simulink model "CAMFC2_Pendulum_Comp_Lewis"  (R2018b)
settings: Solver=ode23  StartTime=0.0  StopTime=40  RelTol=1e-3  EnableMultiTasking=on
InitFcn:
  | constants_CAMFC2_Pendulum_Comp_Lewis
values from neighbouring files (symbols this model uses):
  AN = [     0 1 0 0 ... (first row only)    [constant_CAMFC2_01_WMR01.m]    (also in constant_CAMFC2_04_Comp.m = [     0 1 0 0 1; constant_CAMFC2_04_Quad_03.m; constant_CAMFC2_04_Simple.m; constant_CAMFC2_04_Simple_DoubleIntegrator.m)
  BN = [     1 0 0 0 ... (first row only)    [constant_CAMFC2_01_WMR01.m]    (also in constant_CAMFC2_04_Comp.m = [     0 0 0 0 0; constant_CAMFC2_04_Quad_03.m; constant_CAMFC2_04_Simple.m; constant_CAMFC2_04_Simple_DoubleIntegrator.m)
  Bp = 0.01    [constant_CAMFC2_04_Comp.m]    (also in constant_CAMFC2_04_Simple.m; constant_CAMFC2_04_Simple_DoubleIntegrator.m; constant_CAMFC2_04_Simple_DoubleIntegrator_02.m; constants_CAMFC2_Pendulum_Comp_Lewis.m)
  c = 2.2    [constants_CAMFC2_Pendulum_Comp_Lewis.m]
  Disturb_Freq = 2    [constant_CAMFC2_04_Comp.m]    (also in constant_CAMFC2_04_Simple.m; constant_CAMFC2_04_Simple_DoubleIntegrator.m; constant_CAMFC2_04_Simple_DoubleIntegrator_02.m; constants_CAMFC2_Pendulum_Comp_Lewis.m)
  Disturb_Val = 1    [constant_CAMFC2_04_Comp.m]    (also in constant_CAMFC2_04_Simple.m; constant_CAMFC2_04_Simple_DoubleIntegrator.m; constant_CAMFC2_04_Simple_DoubleIntegrator_02.m; constants_CAMFC2_Pendulum_Comp_Lewis.m)
  DN = [     1 0 0 0 ... (first row only)    [constant_CAMFC2_01_WMR01.m]    (also in constant_CAMFC2_04_Comp.m = [     2 0 0 0 0; constant_CAMFC2_04_Quad_03.m; constant_CAMFC2_04_Simple.m; constant_CAMFC2_04_Simple_DoubleIntegrator.m)
  F = 1.63    [constants_CAMFC2_Pendulum_Comp_Lewis.m]
  ge = 9.81    [constant_CAMFC2_04_Comp.m]    (also in constant_CAMFC2_04_Quad_03.m; constant_CAMFC2_04_Simple.m; constant_CAMFC2_04_Simple_DoubleIntegrator.m; constant_CAMFC2_04_Simple_DoubleIntegrator_02.m)
  Jp = 1    [constant_CAMFC2_04_Comp.m]    (also in constant_CAMFC2_04_Simple.m; constant_CAMFC2_04_Simple_DoubleIntegrator.m; constant_CAMFC2_04_Simple_DoubleIntegrator_02.m; constants_CAMFC2_Pendulum_Comp_Lewis.m)
  k = 1    [constants_CAMFC2_Pendulum_Comp_Lewis.m]
  k_NN = 1    [constants_CAMFC2_Pendulum_Comp_Lewis.m]
  lambda = 10    [constants_CAMFC2_Pendulum_Comp_Lewis.m]
  lp = 0.1    [constant_CAMFC2_04_Comp.m]    (also in constant_CAMFC2_04_Simple.m; constant_CAMFC2_04_Simple_DoubleIntegrator.m; constant_CAMFC2_04_Simple_DoubleIntegrator_02.m; constants_CAMFC2_Pendulum_Comp_Lewis.m)
  Mp = 0.1    [constant_CAMFC2_04_Comp.m]    (also in constant_CAMFC2_04_Simple.m; constant_CAMFC2_04_Simple_DoubleIntegrator.m; constant_CAMFC2_04_Simple_DoubleIntegrator_02.m; constants_CAMFC2_Pendulum_Comp_Lewis.m)
  N = 4    [constant_CAMFC2_01_WMR01.m]    (also in constant_CAMFC2_04_Comp.m = 5; constant_CAMFC2_04_Quad_03.m; constant_CAMFC2_04_Simple.m; constant_CAMFC2_04_Simple_DoubleIntegrator.m)
  n = 4    [constant_CAMFC2_01_WMR01.m]    (also in constant_CAMFC2_04_Comp.m = 2; constant_CAMFC2_04_Quad_03.m = 6; constant_CAMFC2_04_Simple.m = 2; constant_CAMFC2_04_Simple_DoubleIntegrator.m = 2)
  NN = 4    [constants_CAMFC2_Pendulum_Comp_Lewis.m]
  P = diag(p)    [constants_CAMFC2_Pendulum_Comp_Lewis.m]
settings Model: Creator=hp  LastModifiedBy=asafae
settings DataIOCC: LimitDataPoints=on  SaveFormat=Array
settings OptimizationCC: LifeSpan=inf
settings DebuggingCC: UnderspecifiedInitializationDetection=Classic  MergeDetectMultiDrivingBlocksExec=none  SolverPrmCheckMsg=warning  SFUnexpectedBacktrackingDiag=warning  SFNoUnconditionalDefaultTransitionDiag=warning  SFExecutionAtInitializationDiag=none
settings HardwareCC: ProdBitPerPointer=32  ProdBitPerSizeT=32  ProdBitPerPtrDiffT=32  ProdLargestAtomicFloat=None  ProdIntDivRoundTo=Undefined  ProdEndianess=Unspecified  ProdWordSize=32  ProdHWDeviceType=32-bit Generic
settings ModelReferenceCC: PropagateSignalLabelsOutOfModel=off
settings SFSimCC: SimUseLocalCustomCode=off
settings RTWCC: RTWUseLocalCustomCode=off
settings CodeAppCC: StateflowObjectComments=on
settings GRTTargetCC: TargetLangStandard=C89/C90 (ANSI)  GeneratePreprocessorConditionals=Disable all
settings ConfigComp: CovMetricSettings=dw  CovHtmlReporting=on  CovSaveCumulativeToWorkspaceVar=on  CovSaveSingleToWorkspaceVar=on  CovExternalEMLEnable=off

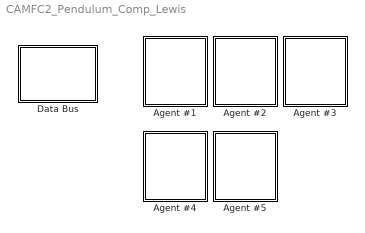
== system CAMFC2_Pendulum_Comp_Lewis ==
  Agent #1 : Subsystem
  Agent #2 : Subsystem
  Agent #3 : Subsystem
  Agent #4 : Subsystem
  Agent #5 : Subsystem
  "Data Bus " : Subsystem

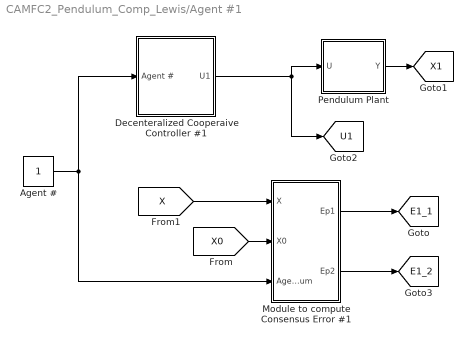
== system CAMFC2_Pendulum_Comp_Lewis/Agent #1 ==
  Agent # : Constant
  Decenteralized Cooperaive Controller #1 : Subsystem
  Module to compute Consensus Error #1 : MATLAB Function  TreatAsAtomicUnit=on
  Pendulum Plant : Subsystem
  tag scope: E1_1=global, E1_2=global, U1=global, X1=global
  wires:
  Agent #/1 -> Module to compute Consensus Error #1/3(Agent_Num), Decenteralized Cooperaive Controller #1/1(Agent #)
  Decenteralized Cooperaive Controller #1/1(U1) -> Pendulum Plant/1(U), [U1]
  [X0] -> Module to compute Consensus Error #1/2(X0)
  [X] -> Module to compute Consensus Error #1/1(X)
  Pendulum Plant/1(Y) -> [X1]
  Module to compute Consensus Error #1/1(Ep1) -> [E1_1]
  Module to compute Consensus Error #1/2(Ep2) -> [E1_2]

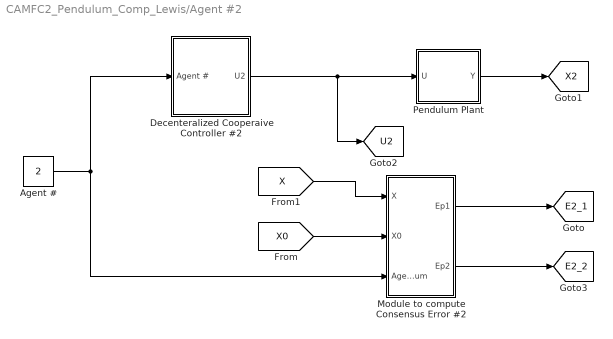
== system CAMFC2_Pendulum_Comp_Lewis/Agent #2 ==
  Agent # : Constant  Value=2
  Decenteralized Cooperaive Controller #2 : Subsystem
  Module to compute Consensus Error #2 : MATLAB Function  TreatAsAtomicUnit=on
  Pendulum Plant : Subsystem
  tag scope: E2_1=global, E2_2=global, U2=global, X2=global
  wires:
  Pendulum Plant/1(Y) -> [X2]
  [X] -> Module to compute Consensus Error #2/1(X)
  [X0] -> Module to compute Consensus Error #2/2(X0)
  Decenteralized Cooperaive Controller #2/1(U2) -> Pendulum Plant/1(U), [U2]
  Agent #/1 -> Decenteralized Cooperaive Controller #2/1(Agent #), Module to compute Consensus Error #2/3(Agent_Num)
  Module to compute Consensus Error #2/1(Ep1) -> [E2_1]
  Module to compute Consensus Error #2/2(Ep2) -> [E2_2]

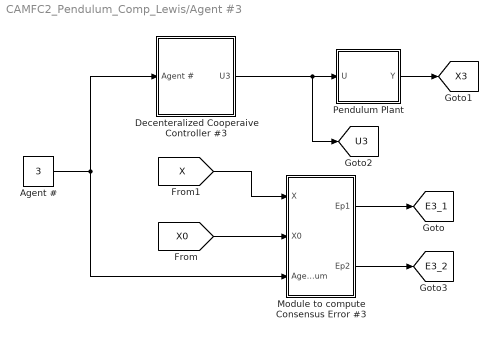
== system CAMFC2_Pendulum_Comp_Lewis/Agent #3 ==
  Agent # : Constant  Value=3
  Decenteralized Cooperaive Controller #3 : Subsystem
  Module to compute Consensus Error #3 : MATLAB Function  TreatAsAtomicUnit=on
  Pendulum Plant : Subsystem
  tag scope: E3_1=global, E3_2=global, U3=global, X3=global
  wires:
  Module to compute Consensus Error #3/2(Ep2) -> [E3_2]
  Module to compute Consensus Error #3/1(Ep1) -> [E3_1]
  Agent #/1 -> Module to compute Consensus Error #3/3(Agent_Num), Decenteralized Cooperaive Controller #3/1(Agent #)
  Decenteralized Cooperaive Controller #3/1(U3) -> Pendulum Plant/1(U), [U3]
  [X0] -> Module to compute Consensus Error #3/2(X0)
  [X] -> Module to compute Consensus Error #3/1(X)
  Pendulum Plant/1(Y) -> [X3]

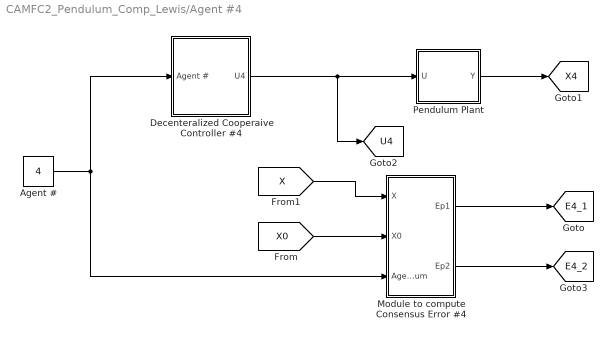
== system CAMFC2_Pendulum_Comp_Lewis/Agent #4 ==
  Agent # : Constant  Value=4
  Decenteralized Cooperaive Controller #4 : Subsystem
  Module to compute Consensus Error #4 : MATLAB Function  TreatAsAtomicUnit=on
  Pendulum Plant : Subsystem
  tag scope: E4_1=global, E4_2=global, U4=global, X4=global
  wires:
  Pendulum Plant/1(Y) -> [X4]
  [X] -> Module to compute Consensus Error #4/1(X)
  [X0] -> Module to compute Consensus Error #4/2(X0)
  Decenteralized Cooperaive Controller #4/1(U4) -> Pendulum Plant/1(U), [U4]
  Agent #/1 -> Decenteralized Cooperaive Controller #4/1(Agent #), Module to compute Consensus Error #4/3(Agent_Num)
  Module to compute Consensus Error #4/1(Ep1) -> [E4_1]
  Module to compute Consensus Error #4/2(Ep2) -> [E4_2]

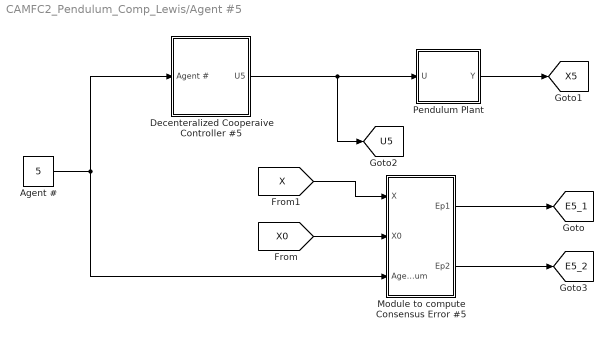
== system CAMFC2_Pendulum_Comp_Lewis/Agent #5 ==
  Agent # : Constant  Value=5
  Decenteralized Cooperaive Controller #5 : Subsystem
  Module to compute Consensus Error #5 : MATLAB Function  TreatAsAtomicUnit=on
  Pendulum Plant : Subsystem
  tag scope: E5_1=global, E5_2=global, U5=global, X5=global
  wires:
  Module to compute Consensus Error #5/2(Ep2) -> [E5_2]
  Module to compute Consensus Error #5/1(Ep1) -> [E5_1]
  Agent #/1 -> Module to compute Consensus Error #5/3(Agent_Num), Decenteralized Cooperaive Controller #5/1(Agent #)
  Decenteralized Cooperaive Controller #5/1(U5) -> Pendulum Plant/1(U), [U5]
  [X0] -> Module to compute Consensus Error #5/2(X0)
  [X] -> Module to compute Consensus Error #5/1(X)
  Pendulum Plant/1(Y) -> [X5]

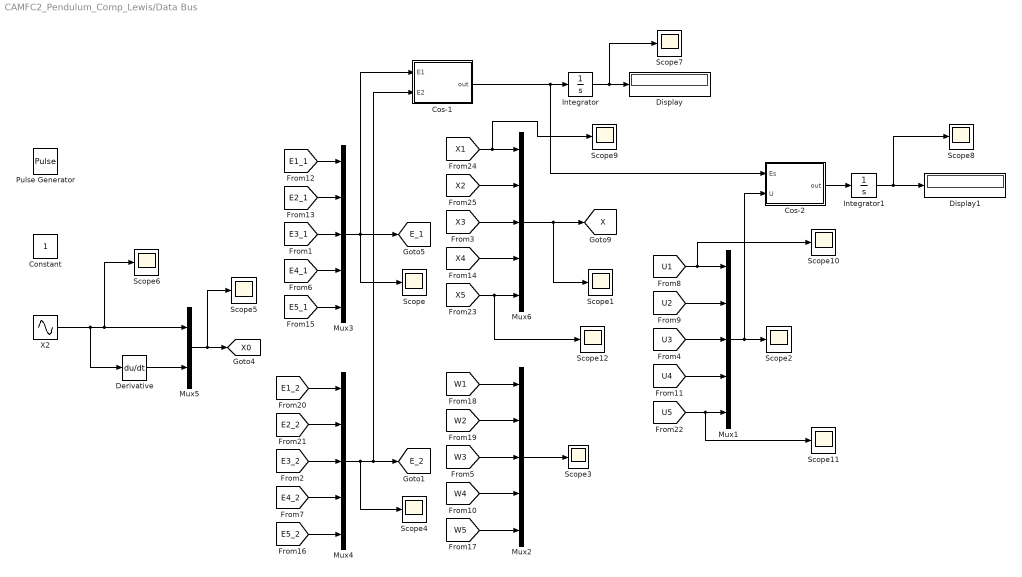
== system CAMFC2_Pendulum_Comp_Lewis/Data Bus  ==
  Constant : Constant
  Cos-1 : MATLAB Function  TreatAsAtomicUnit=on
  Cos-2 : MATLAB Function  TreatAsAtomicUnit=on
  Derivative : Derivative
  Display : Display
  Display1 : Display
  Integrator : Integrator
  Integrator1 : Integrator
  Mux{1..4,6} (5 alike) : Mux  Inputs=5
  Mux5 : Mux  Inputs=2
  Pulse Generator : DiscretePulseGenerator  PulseType=Time based  Amplitude=2  Period=20  PulseWidth=50
  Scope{,1..12} (13 alike) : Scope
  X2 : Sin  Amplitude=3  Frequency=0.5  SampleTime=0
  tag scope: E_1=global, E_2=global, X0=global, X=global
  wires:
  [E2_1] -> Mux3/2
  [E1_1] -> Mux3/1
  Mux3/1 -> Cos-1/1(E1), Scope/1, [E_1]
  [X2] -> Mux6/2
  [X1] -> Scope9/1, Mux6/1
  Mux6/1 -> Scope1/1, [X]
  [U2] -> Mux1/2
  [U1] -> Scope10/1, Mux1/1
  [W2] -> Mux2/2
  [W1] -> Mux2/1
  Mux2/1 -> Scope3/1
  [E2_2] -> Mux4/2
  [E1_2] -> Mux4/1
  Mux4/1 -> Cos-1/2(E2), [E_2], Scope4/1
  Mux5/1 -> Scope5/1, [X0]
  X2/1 -> Derivative/1, Scope6/1, Mux5/1
  Derivative/1 -> Mux5/2
  [E3_1] -> Mux3/3
  [E3_2] -> Mux4/3
  [X3] -> Mux6/3
  [U3] -> Mux1/3
  [W3] -> Mux2/3
  [E4_1] -> Mux3/4
  [E4_2] -> Mux4/4
  [W4] -> Mux2/4
  [U4] -> Mux1/4
  [X4] -> Mux6/4
  [E5_1] -> Mux3/5
  [E5_2] -> Mux4/5
  [W5] -> Mux2/5
  [U5] -> Scope11/1, Mux1/5
  [X5] -> Scope12/1, Mux6/5
  Cos-1/1(out) -> Cos-2/1(Es), Integrator/1
  Integrator/1 -> Scope7/1, Display/1
  Integrator1/1 -> Display1/1, Scope8/1
  Cos-2/1(out) -> Integrator1/1
  Mux1/1 -> Cos-2/2(U), Scope2/1

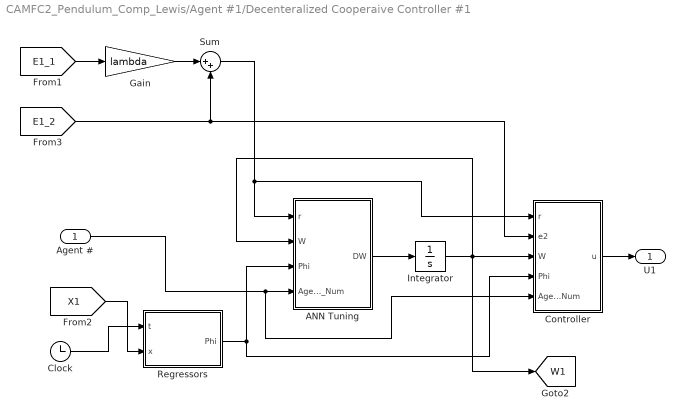
== system CAMFC2_Pendulum_Comp_Lewis/Agent #1/Decenteralized Cooperaive Controller #1 ==
  Agent # : Inport
  ANN Tuning : MATLAB Function  TreatAsAtomicUnit=on
  Clock : Clock
  Controller : MATLAB Function  TreatAsAtomicUnit=on
  Gain : Gain  Gain=lambda
  Integrator : Integrator  InitialCondition=zeros(NN,1)
  Regressors : MATLAB Function  TreatAsAtomicUnit=on
  Sum : Sum  Inputs=|++
  U1 : Outport
  tag scope: W1=global
  wires:
  ANN Tuning/1(DW) -> Integrator/1
  Integrator/1 -> ANN Tuning/2(W), [W1], Controller/3(W)
  Regressors/1(Phi) -> Controller/4(Phi), ANN Tuning/3(Phi)
  Agent #/1 -> Controller/5(Agent_Num), ANN Tuning/4(Agent_Num)
  Controller/1(u) -> U1/1
  Sum/1 -> Controller/1(r), ANN Tuning/1(r)
  [E1_2] -> Sum/2, Controller/2(e2)
  [E1_1] -> Gain/1
  Gain/1 -> Sum/1
  Clock/1 -> Regressors/1(t)
  [X1] -> Regressors/2(x)

== system CAMFC2_Pendulum_Comp_Lewis/Agent #1/Pendulum Plant ==
  U : Inport
  Plant : Subsystem
  Y : Outport
  wires:
  U/1 -> Plant/1(U)
  Plant/1(Y) -> Y/1

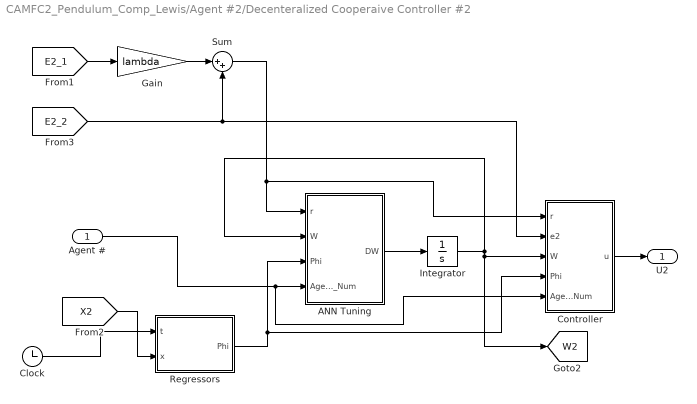
== system CAMFC2_Pendulum_Comp_Lewis/Agent #2/Decenteralized Cooperaive Controller #2 ==
  Agent # : Inport
  ANN Tuning : MATLAB Function  TreatAsAtomicUnit=on
  Clock : Clock
  Controller : MATLAB Function  TreatAsAtomicUnit=on
  Gain : Gain  Gain=lambda
  Integrator : Integrator  InitialCondition=zeros(NN,1)
  Regressors : MATLAB Function  TreatAsAtomicUnit=on
  Sum : Sum  Inputs=|++
  U2 : Outport
  tag scope: W2=global
  wires:
  Gain/1 -> Sum/1
  [E2_1] -> Gain/1
  [E2_2] -> Controller/2(e2), Sum/2
  Sum/1 -> Controller/1(r), ANN Tuning/1(r)
  Controller/1(u) -> U2/1
  Agent #/1 -> Controller/5(Agent_Num), ANN Tuning/4(Agent_Num)
  Regressors/1(Phi) -> Controller/4(Phi), ANN Tuning/3(Phi)
  Integrator/1 -> [W2], Controller/3(W), ANN Tuning/2(W)
  ANN Tuning/1(DW) -> Integrator/1
  Clock/1 -> Regressors/1(t)
  [X2] -> Regressors/2(x)

== system CAMFC2_Pendulum_Comp_Lewis/Agent #2/Pendulum Plant ==
  U : Inport
  Plant : Subsystem
  Y : Outport
  wires:
  U/1 -> Plant/1(U)
  Plant/1(Y) -> Y/1

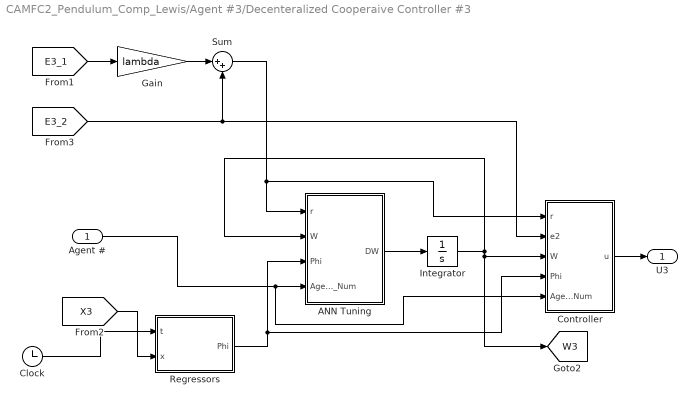
== system CAMFC2_Pendulum_Comp_Lewis/Agent #3/Decenteralized Cooperaive Controller #3 ==
  Agent # : Inport
  ANN Tuning : MATLAB Function  TreatAsAtomicUnit=on
  Clock : Clock
  Controller : MATLAB Function  TreatAsAtomicUnit=on
  Gain : Gain  Gain=lambda
  Integrator : Integrator  InitialCondition=zeros(NN,1)
  Regressors : MATLAB Function  TreatAsAtomicUnit=on
  Sum : Sum  Inputs=|++
  U3 : Outport
  tag scope: W3=global
  wires:
  ANN Tuning/1(DW) -> Integrator/1
  Integrator/1 -> ANN Tuning/2(W), Controller/3(W), [W3]
  Regressors/1(Phi) -> ANN Tuning/3(Phi), Controller/4(Phi)
  Agent #/1 -> ANN Tuning/4(Agent_Num), Controller/5(Agent_Num)
  Controller/1(u) -> U3/1
  Sum/1 -> ANN Tuning/1(r), Controller/1(r)
  [E3_2] -> Sum/2, Controller/2(e2)
  [E3_1] -> Gain/1
  Gain/1 -> Sum/1
  Clock/1 -> Regressors/1(t)
  [X3] -> Regressors/2(x)

== system CAMFC2_Pendulum_Comp_Lewis/Agent #3/Pendulum Plant ==
  U : Inport
  Plant : Subsystem
  Y : Outport
  wires:
  U/1 -> Plant/1(U)
  Plant/1(Y) -> Y/1

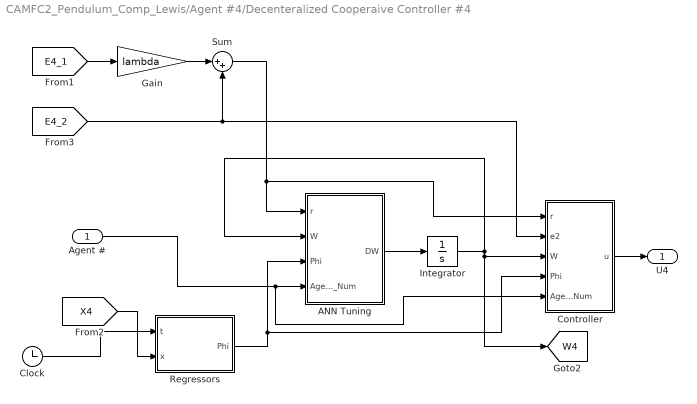
== system CAMFC2_Pendulum_Comp_Lewis/Agent #4/Decenteralized Cooperaive Controller #4 ==
  Agent # : Inport
  ANN Tuning : MATLAB Function  TreatAsAtomicUnit=on
  Clock : Clock
  Controller : MATLAB Function  TreatAsAtomicUnit=on
  Gain : Gain  Gain=lambda
  Integrator : Integrator  InitialCondition=zeros(NN,1)
  Regressors : MATLAB Function  TreatAsAtomicUnit=on
  Sum : Sum  Inputs=|++
  U4 : Outport
  tag scope: W4=global
  wires:
  Gain/1 -> Sum/1
  [E4_1] -> Gain/1
  [E4_2] -> Controller/2(e2), Sum/2
  Sum/1 -> Controller/1(r), ANN Tuning/1(r)
  Controller/1(u) -> U4/1
  Agent #/1 -> Controller/5(Agent_Num), ANN Tuning/4(Agent_Num)
  Regressors/1(Phi) -> Controller/4(Phi), ANN Tuning/3(Phi)
  Integrator/1 -> [W4], Controller/3(W), ANN Tuning/2(W)
  ANN Tuning/1(DW) -> Integrator/1
  Clock/1 -> Regressors/1(t)
  [X4] -> Regressors/2(x)

== system CAMFC2_Pendulum_Comp_Lewis/Agent #4/Pendulum Plant ==
  U : Inport
  Plant : Subsystem
  Y : Outport
  wires:
  U/1 -> Plant/1(U)
  Plant/1(Y) -> Y/1

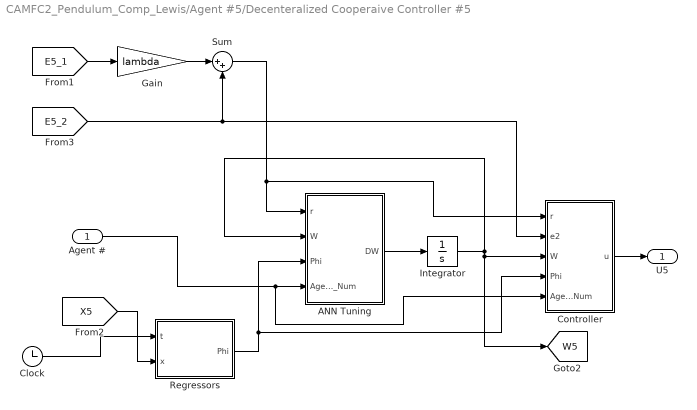
== system CAMFC2_Pendulum_Comp_Lewis/Agent #5/Decenteralized Cooperaive Controller #5 ==
  Agent # : Inport
  ANN Tuning : MATLAB Function  TreatAsAtomicUnit=on
  Clock : Clock
  Controller : MATLAB Function  TreatAsAtomicUnit=on
  Gain : Gain  Gain=lambda
  Integrator : Integrator  InitialCondition=zeros(NN,1)
  Regressors : MATLAB Function  TreatAsAtomicUnit=on
  Sum : Sum  Inputs=|++
  U5 : Outport
  tag scope: W5=global
  wires:
  ANN Tuning/1(DW) -> Integrator/1
  Integrator/1 -> ANN Tuning/2(W), Controller/3(W), [W5]
  Regressors/1(Phi) -> ANN Tuning/3(Phi), Controller/4(Phi)
  Agent #/1 -> ANN Tuning/4(Agent_Num), Controller/5(Agent_Num)
  Controller/1(u) -> U5/1
  Sum/1 -> ANN Tuning/1(r), Controller/1(r)
  [E5_2] -> Sum/2, Controller/2(e2)
  [E5_1] -> Gain/1
  Gain/1 -> Sum/1
  Clock/1 -> Regressors/1(t)
  [X5] -> Regressors/2(x)

== system CAMFC2_Pendulum_Comp_Lewis/Agent #5/Pendulum Plant ==
  U : Inport
  Plant : Subsystem
  Y : Outport
  wires:
  U/1 -> Plant/1(U)
  Plant/1(Y) -> Y/1

== system CAMFC2_Pendulum_Comp_Lewis/Agent #1/Pendulum Plant/Plant ==
  U : Inport
  Clock : Clock
  Integrator : Integrator
  Integrator1 : Integrator
  Mux : Mux  Inputs=2
  Plant : MATLAB Function  TreatAsAtomicUnit=on
  Scope3 : Scope
  Y : Outport
  wires:
  Plant/1(Dx1) -> Integrator/1
  Integrator/1 -> Plant/1(x1), Mux/1
  Integrator1/1 -> Plant/2(x2), Mux/2
  U/1 -> Plant/3(u)
  Plant/2(Dx2) -> Integrator1/1
  Clock/1 -> Plant/4(t)
  Mux/1 -> Y/1, Scope3/1

== system CAMFC2_Pendulum_Comp_Lewis/Agent #2/Pendulum Plant/Plant ==
  U : Inport
  Clock : Clock
  Integrator : Integrator  InitialCondition=-0.5
  Integrator1 : Integrator
  Mux : Mux  Inputs=2
  Plant : MATLAB Function  TreatAsAtomicUnit=on
  Scope3 : Scope
  Y : Outport
  wires:
  Plant/1(Dx1) -> Integrator/1
  Integrator/1 -> Plant/1(x1), Mux/1
  Integrator1/1 -> Plant/2(x2), Mux/2
  U/1 -> Plant/3(u)
  Plant/2(Dx2) -> Integrator1/1
  Clock/1 -> Plant/4(t)
  Mux/1 -> Y/1, Scope3/1

== system CAMFC2_Pendulum_Comp_Lewis/Agent #3/Pendulum Plant/Plant ==
  U : Inport
  Clock : Clock
  Integrator : Integrator  InitialCondition=+0.5
  Integrator1 : Integrator
  Mux : Mux  Inputs=2
  Plant : MATLAB Function  TreatAsAtomicUnit=on
  Scope3 : Scope
  Y : Outport
  wires:
  Plant/1(Dx1) -> Integrator/1
  Integrator/1 -> Plant/1(x1), Mux/1
  Integrator1/1 -> Plant/2(x2), Mux/2
  U/1 -> Plant/3(u)
  Plant/2(Dx2) -> Integrator1/1
  Clock/1 -> Plant/4(t)
  Mux/1 -> Y/1, Scope3/1

== system CAMFC2_Pendulum_Comp_Lewis/Agent #4/Pendulum Plant/Plant ==
  U : Inport
  Clock : Clock
  Integrator : Integrator  InitialCondition=-1
  Integrator1 : Integrator
  Mux : Mux  Inputs=2
  Plant : MATLAB Function  TreatAsAtomicUnit=on
  Scope3 : Scope
  Y : Outport
  wires:
  Plant/1(Dx1) -> Integrator/1
  Integrator/1 -> Plant/1(x1), Mux/1
  Integrator1/1 -> Plant/2(x2), Mux/2
  U/1 -> Plant/3(u)
  Plant/2(Dx2) -> Integrator1/1
  Clock/1 -> Plant/4(t)
  Mux/1 -> Y/1, Scope3/1

== system CAMFC2_Pendulum_Comp_Lewis/Agent #5/Pendulum Plant/Plant ==
  U : Inport
  Clock : Clock
  Integrator : Integrator  InitialCondition=+1
  Integrator1 : Integrator
  Mux : Mux  Inputs=2
  Plant : MATLAB Function  TreatAsAtomicUnit=on
  Scope3 : Scope
  Y : Outport
  wires:
  Plant/1(Dx1) -> Integrator/1
  Integrator/1 -> Plant/1(x1), Mux/1
  Integrator1/1 -> Plant/2(x2), Mux/2
  U/1 -> Plant/3(u)
  Plant/2(Dx2) -> Integrator1/1
  Clock/1 -> Plant/4(t)
  Mux/1 -> Y/1, Scope3/1

== matlab function CAMFC2_Pendulum_Comp_Lewis/Agent #2/Decenteralized Cooperaive Controller #2/ANN Tuning ==
  data: F parameter; r input; W input; Phi input; DW output; P parameter; DN parameter; BN parameter; k parameter; Agent_Num input
function DW = fcn(F,r,W,Phi, P, DN, BN, k,Agent_Num)

DW = -F * Phi * r' * P(Agent_Num,Agent_Num) * (DN(Agent_Num,Agent_Num)+BN(Agent_Num,Agent_Num)) - k * F * W;

end

== matlab function CAMFC2_Pendulum_Comp_Lewis/Agent #2/Decenteralized Cooperaive Controller #2/Controller ==
  data: u output size=1; r input; e2 input; W input; Phi input; Agent_Num input; c parameter; lambda parameter; BN parameter; DN parameter
function u = fcn(r,e2,W,Phi,Agent_Num, c, lambda, BN, DN)

u = (c*r) - (W' * Phi) + ( lambda / (DN(Agent_Num,Agent_Num)+BN(Agent_Num,Agent_Num)) * (e2) );

end

== matlab function CAMFC2_Pendulum_Comp_Lewis/Agent #2/Decenteralized Cooperaive Controller #2/Regressors ==
  data: t input; x input; Phi output; k_NN parameter; NN parameter
function Phi = fcn(t,x, k_NN, NN)

Phi = [(1/(1+exp(-k_NN*t)));(1/(1+exp(-k_NN*t)));(1/(1+exp(-k_NN*t)));(1/(1+exp(-k_NN*t)))]; %[1;x(1);(x(1)^2)];%;(x^3)];

end

== matlab function CAMFC2_Pendulum_Comp_Lewis/Agent #2/Module to compute Consensus Error #2 ==
  data: X input; X0 input; Ep1 output; AN parameter; BN parameter; N parameter; n parameter; Agent_Num input; Ep2 output
function [Ep1,Ep2] = fcn(X,X0,AN,BN,N,n,Agent_Num)

Xp1 = zeros(1,N);
Xp2 = zeros(1,N);
for i=1:N
    Xp1(1,i) = X((i-1)*n+1);
    Xp2(1,i) = X((i*n));
end

%% ---------------------------------------------------------------

Xp1_own = Xp1(1,Agent_Num);
Xp2_own = Xp2(1,Agent_Num);

Xp01 = X0(1);
Xp02 = X0(2);

Ep1 = ( BN(Agent_Num,Agent_Num)*(Xp01 - Xp1_own) );
Ep2 = ( BN(Agent_Num,Agent_Num)*(Xp02 - Xp2_own) );

for i=1:N        
    Xp1_other = Xp1(1,i);
    Xp2_other = Xp2(1,i);
    Ep1 = Ep1 + AN(Agent_Num,i)*(Xp1_other - Xp1_own);
    Ep2 = Ep2 + AN(Agent_Num,i)*(Xp2_other - Xp2_own);
end

end

== matlab function CAMFC2_Pendulum_Comp_Lewis/Agent #2/Pendulum Plant/Plant/Plant ==
  data: x1 input; Dx1 output; x2 input; Dx2 output; u input; t input; Jp parameter; Bp parameter; Mp parameter; ge parameter; lp parameter; Disturb_Val parameter; Disturb_Freq parameter
function [Dx1,Dx2]  = fcn(x1,x2,u,t,Jp, Bp, Mp, ge, lp, Disturb_Val, Disturb_Freq)

Dx1 = x2;
Dx2 = (1/Jp) * (u - Bp*x2 - Mp*ge*lp*sin(x1) + (Disturb_Val*sin(Disturb_Freq*t)));

end

== matlab function CAMFC2_Pendulum_Comp_Lewis/Agent #3/Decenteralized Cooperaive Controller #3/ANN Tuning ==
  data: F parameter; r input; W input; Phi input; DW output; P parameter; DN parameter; BN parameter; k parameter; Agent_Num input
function DW = fcn(F,r,W,Phi, P, DN, BN, k,Agent_Num)

DW = -F * Phi * r' * P(Agent_Num,Agent_Num) * (DN(Agent_Num,Agent_Num)+BN(Agent_Num,Agent_Num)) - k * F * W;

end

== matlab function CAMFC2_Pendulum_Comp_Lewis/Agent #3/Decenteralized Cooperaive Controller #3/Controller ==
  data: u output size=1; r input; e2 input; W input; Phi input; Agent_Num input; c parameter; lambda parameter; BN parameter; DN parameter
function u = fcn(r,e2,W,Phi,Agent_Num, c, lambda, BN, DN)

u = (c*r) - (W' * Phi) + ( lambda / (DN(Agent_Num,Agent_Num)+BN(Agent_Num,Agent_Num)) * (e2) );

end

== matlab function CAMFC2_Pendulum_Comp_Lewis/Agent #3/Decenteralized Cooperaive Controller #3/Regressors ==
  data: t input; x input; Phi output; k_NN parameter; NN parameter
function Phi = fcn(t,x, k_NN, NN)

Phi = [(1/(1+exp(-k_NN*t)));(1/(1+exp(-k_NN*t)));(1/(1+exp(-k_NN*t)));(1/(1+exp(-k_NN*t)))]; %[1;x(1);(x(1)^2)];%;(x^3)];

end

== matlab function CAMFC2_Pendulum_Comp_Lewis/Agent #3/Module to compute Consensus Error #3 ==
  data: X input; X0 input; Ep1 output; AN parameter; BN parameter; N parameter; n parameter; Agent_Num input; Ep2 output
function [Ep1,Ep2] = fcn(X,X0,AN,BN,N,n,Agent_Num)

Xp1 = zeros(1,N);
Xp2 = zeros(1,N);
for i=1:N
    Xp1(1,i) = X((i-1)*n+1);
    Xp2(1,i) = X((i*n));
end

%% ---------------------------------------------------------------

Xp1_own = Xp1(1,Agent_Num);
Xp2_own = Xp2(1,Agent_Num);

Xp01 = X0(1);
Xp02 = X0(2);

Ep1 = ( BN(Agent_Num,Agent_Num)*(Xp01 - Xp1_own) );
Ep2 = ( BN(Agent_Num,Agent_Num)*(Xp02 - Xp2_own) );

for i=1:N        
    Xp1_other = Xp1(1,i);
    Xp2_other = Xp2(1,i);
    Ep1 = Ep1 + AN(Agent_Num,i)*(Xp1_other - Xp1_own);
    Ep2 = Ep2 + AN(Agent_Num,i)*(Xp2_other - Xp2_own);
end

end

== matlab function CAMFC2_Pendulum_Comp_Lewis/Agent #3/Pendulum Plant/Plant/Plant ==
  data: x1 input; Dx1 output; x2 input; Dx2 output; u input; t input; Jp parameter; Bp parameter; Mp parameter; ge parameter; lp parameter; Disturb_Val parameter; Disturb_Freq parameter
function [Dx1,Dx2]  = fcn(x1,x2,u,t,Jp, Bp, Mp, ge, lp, Disturb_Val, Disturb_Freq)

Dx1 = x2;
Dx2 = (1/Jp) * (u - Bp*x2 - Mp*ge*lp*sin(x1) + (Disturb_Val*sin(Disturb_Freq*t)));

end

== matlab function CAMFC2_Pendulum_Comp_Lewis/Agent #4/Decenteralized Cooperaive Controller #4/ANN Tuning ==
  data: F parameter; r input; W input; Phi input; DW output; P parameter; DN parameter; BN parameter; k parameter; Agent_Num input
function DW = fcn(F,r,W,Phi, P, DN, BN, k,Agent_Num)

DW = -F * Phi * r' * P(Agent_Num,Agent_Num) * (DN(Agent_Num,Agent_Num)+BN(Agent_Num,Agent_Num)) - k * F * W;

end

== matlab function CAMFC2_Pendulum_Comp_Lewis/Agent #4/Decenteralized Cooperaive Controller #4/Controller ==
  data: u output size=1; r input; e2 input; W input; Phi input; Agent_Num input; c parameter; lambda parameter; BN parameter; DN parameter
function u = fcn(r,e2,W,Phi,Agent_Num, c, lambda, BN, DN)

u = (c*r) - (W' * Phi) + ( lambda / (DN(Agent_Num,Agent_Num)+BN(Agent_Num,Agent_Num)) * (e2) );

end

== matlab function CAMFC2_Pendulum_Comp_Lewis/Agent #4/Decenteralized Cooperaive Controller #4/Regressors ==
  data: t input; x input; Phi output; k_NN parameter; NN parameter
function Phi = fcn(t,x, k_NN, NN)

Phi = [(1/(1+exp(-k_NN*t)));(1/(1+exp(-k_NN*t)));(1/(1+exp(-k_NN*t)));(1/(1+exp(-k_NN*t)))]; %[1;x(1);(x(1)^2)];%;(x^3)];

end

== matlab function CAMFC2_Pendulum_Comp_Lewis/Agent #1/Decenteralized Cooperaive Controller #1/Controller ==
  data: u output size=1; r input; e2 input; W input; Phi input; Agent_Num input; c parameter; lambda parameter; BN parameter; DN parameter
function u = fcn(r,e2,W,Phi,Agent_Num, c, lambda, BN, DN)

u = (c*r) - (W' * Phi) + ( lambda / (DN(Agent_Num,Agent_Num)+BN(Agent_Num,Agent_Num)) * e2 );

end

== matlab function CAMFC2_Pendulum_Comp_Lewis/Agent #1/Decenteralized Cooperaive Controller #1/ANN Tuning ==
  data: F parameter; r input; W input; Phi input; DW output; P parameter; DN parameter; BN parameter; k parameter; Agent_Num input
function DW = fcn(F,r,W,Phi, P, DN, BN, k,Agent_Num)

DW = -F * Phi * r' * P(Agent_Num,Agent_Num) * (DN(Agent_Num,Agent_Num)+BN(Agent_Num,Agent_Num)) - k * F * W;

end

== matlab function CAMFC2_Pendulum_Comp_Lewis/Agent #1/Decenteralized Cooperaive Controller #1/Regressors ==
  data: t input; x input; Phi output; k_NN parameter; NN parameter
function Phi = fcn(t,x, k_NN, NN)

Phi = [(1/(1+exp(-k_NN*t)));(1/(1+exp(-k_NN*t)));(1/(1+exp(-k_NN*t)));(1/(1+exp(-k_NN*t)))]; %[1;x(1);(x(1)^2)];%;(x^3)];

end

== matlab function CAMFC2_Pendulum_Comp_Lewis/Agent #1/Pendulum Plant/Plant/Plant ==
  data: x1 input; Dx1 output; x2 input; Dx2 output; u input; t input; Jp parameter; Bp parameter; Mp parameter; ge parameter; lp parameter; Disturb_Val parameter; Disturb_Freq parameter
function [Dx1,Dx2]  = fcn(x1,x2,u,t,Jp, Bp, Mp, ge, lp, Disturb_Val, Disturb_Freq)

Dx1 = x2;
Dx2 = (1/Jp) * (u - Bp*x2 - Mp*ge*lp*sin(x1) + (Disturb_Val*sin(Disturb_Freq*t)));

end

== matlab function CAMFC2_Pendulum_Comp_Lewis/Agent #4/Module to compute Consensus Error #4 ==
  data: X input; X0 input; Ep1 output; AN parameter; BN parameter; N parameter; n parameter; Agent_Num input; Ep2 output
function [Ep1,Ep2] = fcn(X,X0,AN,BN,N,n,Agent_Num)

Xp1 = zeros(1,N);
Xp2 = zeros(1,N);
for i=1:N
    Xp1(1,i) = X((i-1)*n+1);
    Xp2(1,i) = X((i*n));
end

%% ---------------------------------------------------------------

Xp1_own = Xp1(1,Agent_Num);
Xp2_own = Xp2(1,Agent_Num);

Xp01 = X0(1);
Xp02 = X0(2);

Ep1 = ( BN(Agent_Num,Agent_Num)*(Xp01 - Xp1_own) );
Ep2 = ( BN(Agent_Num,Agent_Num)*(Xp02 - Xp2_own) );

for i=1:N        
    Xp1_other = Xp1(1,i);
    Xp2_other = Xp2(1,i);
    Ep1 = Ep1 + AN(Agent_Num,i)*(Xp1_other - Xp1_own);
    Ep2 = Ep2 + AN(Agent_Num,i)*(Xp2_other - Xp2_own);
end

end

== matlab function CAMFC2_Pendulum_Comp_Lewis/Agent #1/Module to compute Consensus Error #1 ==
  data: X input; X0 input; Ep1 output; AN parameter; BN parameter; N parameter; n parameter; Agent_Num input; Ep2 output
function [Ep1,Ep2] = fcn(X,X0,AN,BN,N,n,Agent_Num)

Xp1 = zeros(1,N);
Xp2 = zeros(1,N);
for i=1:N
    Xp1(1,i) = X((i-1)*n+1);
    Xp2(1,i) = X((i*n));
end

%% ---------------------------------------------------------------

Xp1_own = Xp1(1,Agent_Num);
Xp2_own = Xp2(1,Agent_Num);

Xp01 = X0(1);
Xp02 = X0(2);

Ep1 = ( BN(Agent_Num,Agent_Num)*(Xp01 - Xp1_own) );
Ep2 = ( BN(Agent_Num,Agent_Num)*(Xp02 - Xp2_own) );

for i=1:N        
    Xp1_other = Xp1(1,i);
    Xp2_other = Xp2(1,i);
    Ep1 = Ep1 + AN(Agent_Num,i)*(Xp1_other - Xp1_own);
    Ep2 = Ep2 + AN(Agent_Num,i)*(Xp2_other - Xp2_own);
end

end

== matlab function CAMFC2_Pendulum_Comp_Lewis/Agent #4/Pendulum Plant/Plant/Plant ==
  data: x1 input; Dx1 output; x2 input; Dx2 output; u input; t input; Jp parameter; Bp parameter; Mp parameter; ge parameter; lp parameter; Disturb_Val parameter; Disturb_Freq parameter
function [Dx1,Dx2]  = fcn(x1,x2,u,t,Jp, Bp, Mp, ge, lp, Disturb_Val, Disturb_Freq)

Dx1 = x2;
Dx2 = (1/Jp) * (u - Bp*x2 - Mp*ge*lp*sin(x1) + (Disturb_Val*sin(Disturb_Freq*t)));

end

== matlab function CAMFC2_Pendulum_Comp_Lewis/Agent #5/Decenteralized Cooperaive Controller #5/ANN Tuning ==
  data: F parameter; r input; W input; Phi input; DW output; P parameter; DN parameter; BN parameter; k parameter; Agent_Num input
function DW = fcn(F,r,W,Phi, P, DN, BN, k,Agent_Num)

DW = -F * Phi * r' * P(Agent_Num,Agent_Num) * (DN(Agent_Num,Agent_Num)+BN(Agent_Num,Agent_Num)) - k * F * W;

end

== matlab function CAMFC2_Pendulum_Comp_Lewis/Agent #5/Decenteralized Cooperaive Controller #5/Controller ==
  data: u output size=1; r input; e2 input; W input; Phi input; Agent_Num input; c parameter; lambda parameter; BN parameter; DN parameter
function u = fcn(r,e2,W,Phi,Agent_Num, c, lambda, BN, DN)

u = (c*r) - (W' * Phi) + ( lambda / (DN(Agent_Num,Agent_Num)+BN(Agent_Num,Agent_Num)) * (e2) );

end

== matlab function CAMFC2_Pendulum_Comp_Lewis/Agent #5/Decenteralized Cooperaive Controller #5/Regressors ==
  data: t input; x input; Phi output; k_NN parameter; NN parameter
function Phi = fcn(t,x, k_NN, NN)

Phi = [(1/(1+exp(-k_NN*t)));(1/(1+exp(-k_NN*t)));(1/(1+exp(-k_NN*t)));(1/(1+exp(-k_NN*t)))]; %[1;x(1);(x(1)^2)];%;(x^3)];

end

== matlab function CAMFC2_Pendulum_Comp_Lewis/Agent #5/Module to compute Consensus Error #5 ==
  data: X input; X0 input; Ep1 output; AN parameter; BN parameter; N parameter; n parameter; Agent_Num input; Ep2 output
function [Ep1,Ep2] = fcn(X,X0,AN,BN,N,n,Agent_Num)

Xp1 = zeros(1,N);
Xp2 = zeros(1,N);
for i=1:N
    Xp1(1,i) = X((i-1)*n+1);
    Xp2(1,i) = X((i*n));
end

%% ---------------------------------------------------------------

Xp1_own = Xp1(1,Agent_Num);
Xp2_own = Xp2(1,Agent_Num);

Xp01 = X0(1);
Xp02 = X0(2);

Ep1 = ( BN(Agent_Num,Agent_Num)*(Xp01 - Xp1_own) );
Ep2 = ( BN(Agent_Num,Agent_Num)*(Xp02 - Xp2_own) );

for i=1:N        
    Xp1_other = Xp1(1,i);
    Xp2_other = Xp2(1,i);
    Ep1 = Ep1 + AN(Agent_Num,i)*(Xp1_other - Xp1_own);
    Ep2 = Ep2 + AN(Agent_Num,i)*(Xp2_other - Xp2_own);
end

end

== matlab function CAMFC2_Pendulum_Comp_Lewis/Agent #5/Pendulum Plant/Plant/Plant ==
  data: x1 input; Dx1 output; x2 input; Dx2 output; u input; t input; Jp parameter; Bp parameter; Mp parameter; ge parameter; lp parameter; Disturb_Val parameter; Disturb_Freq parameter
function [Dx1,Dx2]  = fcn(x1,x2,u,t,Jp, Bp, Mp, ge, lp, Disturb_Val, Disturb_Freq)

Dx1 = x2;
Dx2 = (1/Jp) * (u - Bp*x2 - Mp*ge*lp*sin(x1) + (Disturb_Val*sin(Disturb_Freq*t)));

end

== matlab function CAMFC2_Pendulum_Comp_Lewis/Data Bus /Cos-1 ==
  data: E1 input; out output; E2 input
function out = fcn(E1,E2)

out = E1'*E1; % + E2'*E2;

end

== matlab function CAMFC2_Pendulum_Comp_Lewis/Data Bus /Cos-2 ==
  data: Es input; out output; U input
function out = fcn(Es,U)

out = Es + U'*U;

end
